simulink model "check_modelcompare_drive"  (R2018b)
settings: configuration reference "Physics" (kept outside this file)
undefined symbols (not defined in the file or in its folder): brake_param, veh_param, x0_positionstates
libraries: simulink x2
settings Model: DataDictionary=check_modelcompare.sldd  OrderedModelArguments=off  Creator=wischnewski  LastModifiedBy=ga25xiw

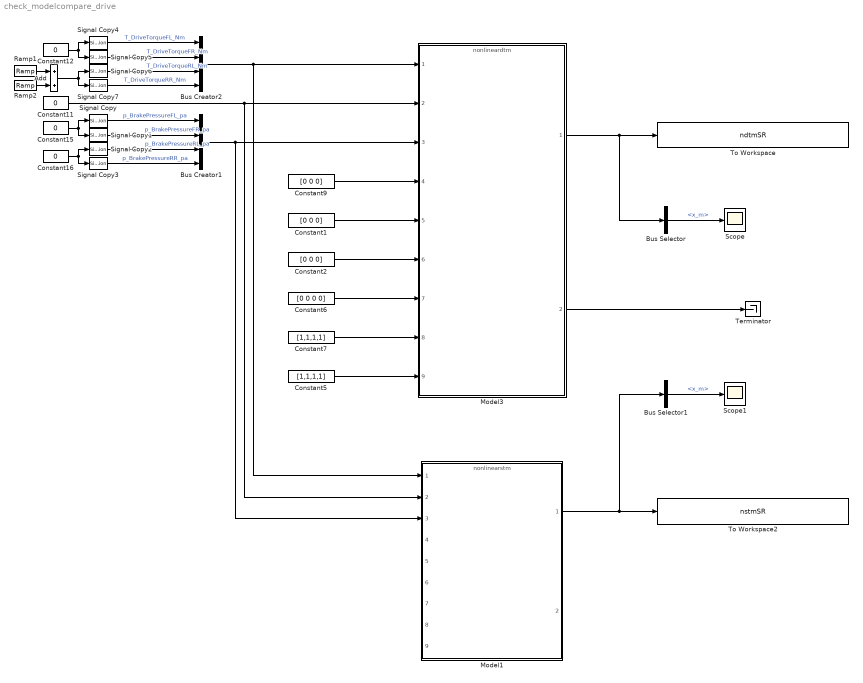
== system check_modelcompare_drive ==
  Add : Sum
  Bus Creator1 : BusCreator  Inputs=4  OutDataTypeStr=Bus: BrakePressure_Pa
  Bus Creator2 : BusCreator  Inputs=4  OutDataTypeStr=Bus: DriveTorque_Nm
  Bus Selector : BusSelector  OutputSignals=x_m
  Bus Selector1 : BusSelector  OutputSignals=x_m
  Constant1 : Constant  Value=[0 0 0]
  Constant{11..12,15..16} (4 alike) : Constant  Value=0
  Constant2 : Constant  Value=[0 0 0]
  Constant5 : Constant  Value=[1,1,1,1]
  Constant6 : Constant  Value=[0 0 0 0]
  Constant7 : Constant  Value=[1,1,1,1]
  Constant9 : Constant  Value=[0 0 0]
  Model1 : ModelReference  ModelNameDialog=nonlinearstm.slx  ParameterArgumentNames=brake_param,veh_param,x0_positionstates  ParameterArgumentValues=brake_param,veh_param,[0,0,-pi/2]  UsingDefaultArgumentValue=0,0,0  SimulationMode=Normal  ModelReferenceVersion=1.335
  Model3 : ModelReference  ModelNameDialog=nonlineardtm  ParameterArgumentNames=x0_vehiclepose  ParameterArgumentValues=[0,0,-pi/2]  UsingDefaultArgumentValue=0  SimulationMode=Normal  ModelReferenceVersion=1.633
  Ramp1 : simulink/Sources/Ramp  slope=50  start=20  InitialOutput=0
  Ramp2 : simulink/Sources/Ramp  slope=-50  start=30  InitialOutput=0
  Scope : Scope
  Scope1 : Scope
  Signal Copy{,1..7} (8 alike) : SignalConversion  OverrideOpt=off
  Terminator : Terminator
  To Workspace : ToWorkspace  VariableName=ndtmSR  SaveFormat=Timeseries  SampleTime=-1
  To Workspace2 : ToWorkspace  VariableName=nstmSR  SaveFormat=Timeseries  SampleTime=-1
  wires:
  Model3/1 -> Bus Selector/1, To Workspace/1
  Constant9/1 -> Model3/4
  Constant1/1 -> Model3/5
  Constant2/1 -> Model3/6
  Constant5/1 -> Model3/9
  Constant6/1 -> Model3/7
  Model3/2 -> Terminator/1
  Ramp1/1 -> Add/1
  Ramp2/1 -> Add/2
  Model1/1 -> Bus Selector1/1, To Workspace2/1
  Constant7/1 -> Model3/8
  Signal Copy2/1 -> Bus Creator1/3  "p_BrakePressureRL_pa"
  Add/1 -> Signal Copy7/1, Signal Copy6/1
  Signal Copy/1 -> Bus Creator1/1  "p_BrakePressureFL_pa"
  Signal Copy1/1 -> Bus Creator1/2  "p_BrakePressureFR_pa"
  Bus Creator1/1 -> Model1/3, Model3/3
  Constant11/1 -> Model1/2, Model3/2
  Bus Creator2/1 -> Model1/1, Model3/1
  Signal Copy5/1 -> Bus Creator2/2  "T_DriveTorqueFR_Nm"
  Signal Copy7/1 -> Bus Creator2/4  "T_DriveTorqueRR_Nm"
  Signal Copy4/1 -> Bus Creator2/1  "T_DriveTorqueFL_Nm"
  Signal Copy6/1 -> Bus Creator2/3  "T_DriveTorqueRL_Nm"
  Constant16/1 -> Signal Copy3/1, Signal Copy2/1
  Signal Copy3/1 -> Bus Creator1/4  "p_BrakePressureRR_pa"
  Constant12/1 -> Signal Copy4/1, Signal Copy5/1
  Constant15/1 -> Signal Copy1/1, Signal Copy/1
  Bus Selector/1 -> Scope/1  "<x_m>"
  Bus Selector1/1 -> Scope1/1  "<x_m>"
